simulink model "Copy_of_VTOLTiltrotor"  (R2024a)
settings: configuration reference "VTOLConfiguration" (kept outside this file)
undefined symbols (not defined in the file): airspeed, Battery, BCE12, BCE_Set_init, BMS_Controller_State, C, Cell10_P, Cell11_P, Cell12_P, Cell1_N, Cell1_P, Cell2_P, Cell3_P, Cell4_P, Cell5_P, Cell6_P, Cell7_P, Cell8_P, Cell9_P, Cell_Temperatures, Cell_Voltages, Charging_State, CityMission, control, controlParams, ControlSampleTime, CriticalTiltAngle, currentFactor, CV_Gain, ddx, ddy, ddz, Device_01, DiscIntNeverNeededParam, dx, dy, dz, Earth, env, F, F28379D_ADC_MaxCount, F28379D_ADC_Vmax, FixedWingMission, flightState, Foc_Ki_IxTcpu, Foc_Ki_S, Foc_Kp_I, Foc_Kp_S, fractalcoef, FSState, FWControlParams, HoverMission, I_cc, Ia_offset, Ib_offset, iniRoll, initPitch, iniYaw, IO334, IO334_DAC_Vmax ... (+55)
libraries: slrealtimeethercatlib x109, simulink x81, fl_lib x65, slpidlib x49, mcbcontrolslib x48, nesl_utility x43, speedgoatlib_hdlCoder_IO3xx x31, canmsglib x17, slrealtimeutilitieslib x13, mcbhdlplantlib x13, speedgoatlib_IO611 x12, dspstat3 x12
(part 5 of 20)

== system Copy_of_VTOLTiltrotor/Motor Control/Controller1/Controller_MIL ==
  Iab : Inport
  QAE_MIL_fbk : Inport  Port=2
  EnablePWM : Inport  Port=3
  Closed_Loop_FOC : Inport  Port=4
  Speed_CMD_RPM : Inport  Port=5
  Controller_Parameters : Inport  Port=6
  Bus Creator : BusCreator  Inputs=5
  Bus Selector : BusSelector  OutputSignals=Ia_offset,Ib_offset,Kp_S,Ki_S,Kp_I,Ki_IxTcpu
  Constant : Constant  Value=0  OutDataTypeStr=single  SampleTime=Ts_CPU
  Constant4 : Constant
  Data Type Conversion : DataTypeConversion  SaturateOnIntegerOverflow=off  RndMeth=Floor
  Data Type Conversion1 : DataTypeConversion  OutDataTypeStr=double  SaturateOnIntegerOverflow=off  RndMeth=Floor
  Data Type Conversion2 : DataTypeConversion  OutDataTypeStr=boolean  SaturateOnIntegerOverflow=off  RndMeth=Floor
  Data Type Conversion4 : DataTypeConversion  OutDataTypeStr=boolean  SaturateOnIntegerOverflow=off  RndMeth=Floor
  Data Type Conversion6 : DataTypeConversion  OutDataTypeStr=uint16  RndMeth=Simplest  SaturateOnIntegerOverflow=off
  F28379D ADC : Subsystem
  F28379D Firmware : Subsystem
  IO334 DAC : Subsystem
  Mux : Mux  Inputs=3
  PWM Generation : pwm_cpulib/PWM Generation  f_FPGA=f_FPGA  n_channels=3  sel_scaling=CPU  protection_param=A/B are forced off when A/B are on.  deadband_sec=0  natural_update=At period starts  delay=0  trigger_duration_sec=[1e-6]  trigger_period_start=off  trigger_half_of_the_period=off  trigger_a_on=off  trigger_a_off=off  trigger_b_on=off  trigger_b_off=off  bit_width_pwm_gen=24  invert_a=off  invert_b=off  invert_c=off
      settings: SourceProductName=PWM CPU Library
  PWM Periods : Constant  Value=[1/PWM_frequency 1/PWM_frequency 1/PWM_frequency]  OutDataTypeStr=double  SampleTime=-1
  Rate Transition1 : RateTransition  OutPortSampleTime=Ts_speed
  Rate Transition12 : RateTransition  OutPortSampleTime=Ts_UI
  Rate Transition{2,4..9} (7 alike) : RateTransition  OutPortSampleTime=Ts_CPU
  Rate Transition3 : RateTransition  OutPortSampleTime=Ts_speed
  bias1 : Constant  OutDataTypeStr=boolean  SampleTime=Ts_CPU
  bias3 : Constant  Value=0  OutDataTypeStr=boolean  SampleTime=Ts_CPU
  Simu_config : Outport
  Controller_fbk : Outport  Port=2
  wires:
  bias1/1 -> Bus Creator/1  "PCIe_RC_or_TTL"
  Bus Creator/1 -> Simu_config/1
  Constant4/1 -> Data Type Conversion6/1
  Data Type Conversion/1 -> Bus Creator/4  "PCIe_PWM_Enable"
  Iab/1 -> IO334 DAC/1(Iab)
  IO334 DAC/1(Iab_IO334DAC) -> F28379D ADC/1(Iab_IO334V)  "IabV"
  F28379D ADC/1(Ia_ADC) -> F28379D Firmware/1(Ia_ADC)
  F28379D ADC/2(Ib_ADC) -> F28379D Firmware/2(Ib_ADC)
  QAE_MIL_fbk/1 -> F28379D Firmware/5(QEP_Position_Count)
  Data Type Conversion6/1 -> F28379D Firmware/6(QEP_Index_Latch)
  Bus Selector/3 -> Rate Transition3/1  "<Kp_S>"
  F28379D Firmware/2(PWM_Enable) -> Data Type Conversion/1
  Data Type Conversion2/1 -> F28379D Firmware/11(EnablePWM)
  Data Type Conversion4/1 -> F28379D Firmware/10(EnClosedLoop)
  Bus Selector/4 -> Rate Transition1/1  "<Ki_S>"
  Closed_Loop_FOC/1 -> Rate Transition4/1
  Controller_Parameters/1 -> Bus Selector/1
  Bus Selector/1 -> Rate Transition5/1  "<Ia_offset>"
  Bus Selector/2 -> Rate Transition6/1  "<Ib_offset>"
  Bus Selector/5 -> Rate Transition8/1  "<Kp_I>"
  Bus Selector/6 -> Rate Transition9/1  "<Ki_IxTcpu>"
  EnablePWM/1 -> Rate Transition7/1
  Mux/1 -> Rate Transition12/1
  F28379D Firmware/3(Fbk_CAN) -> Mux/1
  Speed_CMD_RPM/1 -> Rate Transition2/1
  Rate Transition3/1 -> F28379D Firmware/8(Kp_S)
  Rate Transition1/1 -> F28379D Firmware/9(Ki_S)
  Rate Transition5/1 -> F28379D Firmware/3(IaOffset)
  Rate Transition6/1 -> F28379D Firmware/4(IbOffset)
  Rate Transition4/1 -> Data Type Conversion4/1
  Rate Transition7/1 -> Data Type Conversion2/1
  Rate Transition8/1 -> F28379D Firmware/12(Kp_i)
  Rate Transition9/1 -> F28379D Firmware/13(Ki_ixTcpu)
  Rate Transition12/1 -> Controller_fbk/1
  Constant/1 -> Mux/3
  Rate Transition2/1 -> F28379D Firmware/7(SpdCmdRPM), Mux/2
  bias3/1 -> Bus Creator/5  "PCIe_Protocol"
  PWM Periods/1 -> PWM Generation/1
  PWM Generation/1 -> Bus Creator/2  "PCIe_PWM_Config"
  PWM Generation/2 -> Bus Creator/3  "PCIe_PWM_Runtime"
  Data Type Conversion1/1 -> PWM Generation/2
  F28379D Firmware/1(ModWave) -> Data Type Conversion1/1

== system Copy_of_VTOLTiltrotor/Motor Control/Controller2/Controller_MIL ==
  Iab : Inport
  QAE_MIL_fbk : Inport  Port=2
  EnablePWM : Inport  Port=3
  Closed_Loop_FOC : Inport  Port=4
  Speed_CMD_RPM : Inport  Port=5
  Controller_Parameters : Inport  Port=6
  Bus Creator : BusCreator  Inputs=5
  Bus Selector : BusSelector  OutputSignals=Ia_offset,Ib_offset,Kp_S,Ki_S,Kp_I,Ki_IxTcpu
  Constant : Constant  Value=0  OutDataTypeStr=single  SampleTime=Ts_CPU
  Constant4 : Constant
  Data Type Conversion : DataTypeConversion  SaturateOnIntegerOverflow=off  RndMeth=Floor
  Data Type Conversion1 : DataTypeConversion  OutDataTypeStr=double  SaturateOnIntegerOverflow=off  RndMeth=Floor
  Data Type Conversion2 : DataTypeConversion  OutDataTypeStr=boolean  SaturateOnIntegerOverflow=off  RndMeth=Floor
  Data Type Conversion4 : DataTypeConversion  OutDataTypeStr=boolean  SaturateOnIntegerOverflow=off  RndMeth=Floor
  Data Type Conversion6 : DataTypeConversion  OutDataTypeStr=uint16  RndMeth=Simplest  SaturateOnIntegerOverflow=off
  F28379D ADC : Subsystem
  F28379D Firmware : Subsystem
  IO334 DAC : Subsystem
  Mux : Mux  Inputs=3
  PWM Generation : pwm_cpulib/PWM Generation  f_FPGA=f_FPGA  n_channels=3  sel_scaling=CPU  protection_param=A/B are forced off when A/B are on.  deadband_sec=0  natural_update=At period starts  delay=0  trigger_duration_sec=[1e-6]  trigger_period_start=off  trigger_half_of_the_period=off  trigger_a_on=off  trigger_a_off=off  trigger_b_on=off  trigger_b_off=off  bit_width_pwm_gen=24  invert_a=off  invert_b=off  invert_c=off
      settings: SourceProductName=PWM CPU Library
  PWM Periods : Constant  Value=[1/PWM_frequency 1/PWM_frequency 1/PWM_frequency]  OutDataTypeStr=double  SampleTime=-1
  Rate Transition1 : RateTransition  OutPortSampleTime=Ts_speed
  Rate Transition12 : RateTransition  OutPortSampleTime=Ts_UI
  Rate Transition{2,4..9} (7 alike) : RateTransition  OutPortSampleTime=Ts_CPU
  Rate Transition3 : RateTransition  OutPortSampleTime=Ts_speed
  bias1 : Constant  OutDataTypeStr=boolean  SampleTime=Ts_CPU
  bias3 : Constant  Value=0  OutDataTypeStr=boolean  SampleTime=Ts_CPU
  Simu_config : Outport
  Controller_fbk : Outport  Port=2
  wires:
  bias1/1 -> Bus Creator/1  "PCIe_RC_or_TTL"
  Bus Creator/1 -> Simu_config/1
  Constant4/1 -> Data Type Conversion6/1
  Data Type Conversion/1 -> Bus Creator/4  "PCIe_PWM_Enable"
  Iab/1 -> IO334 DAC/1(Iab)
  IO334 DAC/1(Iab_IO334DAC) -> F28379D ADC/1(Iab_IO334V)  "IabV"
  F28379D ADC/1(Ia_ADC) -> F28379D Firmware/1(Ia_ADC)
  F28379D ADC/2(Ib_ADC) -> F28379D Firmware/2(Ib_ADC)
  QAE_MIL_fbk/1 -> F28379D Firmware/5(QEP_Position_Count)
  Data Type Conversion6/1 -> F28379D Firmware/6(QEP_Index_Latch)
  Bus Selector/3 -> Rate Transition3/1  "<Kp_S>"
  F28379D Firmware/2(PWM_Enable) -> Data Type Conversion/1
  Data Type Conversion2/1 -> F28379D Firmware/11(EnablePWM)
  Data Type Conversion4/1 -> F28379D Firmware/10(EnClosedLoop)
  Bus Selector/4 -> Rate Transition1/1  "<Ki_S>"
  Closed_Loop_FOC/1 -> Rate Transition4/1
  Controller_Parameters/1 -> Bus Selector/1
  Bus Selector/1 -> Rate Transition5/1  "<Ia_offset>"
  Bus Selector/2 -> Rate Transition6/1  "<Ib_offset>"
  Bus Selector/5 -> Rate Transition8/1  "<Kp_I>"
  Bus Selector/6 -> Rate Transition9/1  "<Ki_IxTcpu>"
  EnablePWM/1 -> Rate Transition7/1
  Mux/1 -> Rate Transition12/1
  F28379D Firmware/3(Fbk_CAN) -> Mux/1
  Speed_CMD_RPM/1 -> Rate Transition2/1
  Rate Transition3/1 -> F28379D Firmware/8(Kp_S)
  Rate Transition1/1 -> F28379D Firmware/9(Ki_S)
  Rate Transition5/1 -> F28379D Firmware/3(IaOffset)
  Rate Transition6/1 -> F28379D Firmware/4(IbOffset)
  Rate Transition4/1 -> Data Type Conversion4/1
  Rate Transition7/1 -> Data Type Conversion2/1
  Rate Transition8/1 -> F28379D Firmware/12(Kp_i)
  Rate Transition9/1 -> F28379D Firmware/13(Ki_ixTcpu)
  Rate Transition12/1 -> Controller_fbk/1
  Constant/1 -> Mux/3
  Rate Transition2/1 -> F28379D Firmware/7(SpdCmdRPM), Mux/2
  bias3/1 -> Bus Creator/5  "PCIe_Protocol"
  PWM Periods/1 -> PWM Generation/1
  PWM Generation/1 -> Bus Creator/2  "PCIe_PWM_Config"
  PWM Generation/2 -> Bus Creator/3  "PCIe_PWM_Runtime"
  Data Type Conversion1/1 -> PWM Generation/2
  F28379D Firmware/1(ModWave) -> Data Type Conversion1/1

== system Copy_of_VTOLTiltrotor/Motor Control/Controller3/Controller_MIL ==
  Iab : Inport
  QAE_MIL_fbk : Inport  Port=2
  EnablePWM : Inport  Port=3
  Closed_Loop_FOC : Inport  Port=4
  Speed_CMD_RPM : Inport  Port=5
  Controller_Parameters : Inport  Port=6
  Bus Creator : BusCreator  Inputs=5
  Bus Selector : BusSelector  OutputSignals=Ia_offset,Ib_offset,Kp_S,Ki_S,Kp_I,Ki_IxTcpu
  Constant : Constant  Value=0  OutDataTypeStr=single  SampleTime=Ts_CPU
  Constant4 : Constant
  Data Type Conversion : DataTypeConversion  SaturateOnIntegerOverflow=off  RndMeth=Floor
  Data Type Conversion1 : DataTypeConversion  OutDataTypeStr=double  SaturateOnIntegerOverflow=off  RndMeth=Floor
  Data Type Conversion2 : DataTypeConversion  OutDataTypeStr=boolean  SaturateOnIntegerOverflow=off  RndMeth=Floor
  Data Type Conversion4 : DataTypeConversion  OutDataTypeStr=boolean  SaturateOnIntegerOverflow=off  RndMeth=Floor
  Data Type Conversion6 : DataTypeConversion  OutDataTypeStr=uint16  RndMeth=Simplest  SaturateOnIntegerOverflow=off
  F28379D ADC : Subsystem
  F28379D Firmware : Subsystem
  IO334 DAC : Subsystem
  Mux : Mux  Inputs=3
  PWM Generation : pwm_cpulib/PWM Generation  f_FPGA=f_FPGA  n_channels=3  sel_scaling=CPU  protection_param=A/B are forced off when A/B are on.  deadband_sec=0  natural_update=At period starts  delay=0  trigger_duration_sec=[1e-6]  trigger_period_start=off  trigger_half_of_the_period=off  trigger_a_on=off  trigger_a_off=off  trigger_b_on=off  trigger_b_off=off  bit_width_pwm_gen=24  invert_a=off  invert_b=off  invert_c=off
      settings: SourceProductName=PWM CPU Library
  PWM Periods : Constant  Value=[1/PWM_frequency 1/PWM_frequency 1/PWM_frequency]  OutDataTypeStr=double  SampleTime=-1
  Rate Transition1 : RateTransition  OutPortSampleTime=Ts_speed
  Rate Transition12 : RateTransition  OutPortSampleTime=Ts_UI
  Rate Transition{2,4..9} (7 alike) : RateTransition  OutPortSampleTime=Ts_CPU
  Rate Transition3 : RateTransition  OutPortSampleTime=Ts_speed
  bias1 : Constant  OutDataTypeStr=boolean  SampleTime=Ts_CPU
  bias3 : Constant  Value=0  OutDataTypeStr=boolean  SampleTime=Ts_CPU
  Simu_config : Outport
  Controller_fbk : Outport  Port=2
  wires:
  bias1/1 -> Bus Creator/1  "PCIe_RC_or_TTL"
  Bus Creator/1 -> Simu_config/1
  Constant4/1 -> Data Type Conversion6/1
  Data Type Conversion/1 -> Bus Creator/4  "PCIe_PWM_Enable"
  Iab/1 -> IO334 DAC/1(Iab)
  IO334 DAC/1(Iab_IO334DAC) -> F28379D ADC/1(Iab_IO334V)  "IabV"
  F28379D ADC/1(Ia_ADC) -> F28379D Firmware/1(Ia_ADC)
  F28379D ADC/2(Ib_ADC) -> F28379D Firmware/2(Ib_ADC)
  QAE_MIL_fbk/1 -> F28379D Firmware/5(QEP_Position_Count)
  Data Type Conversion6/1 -> F28379D Firmware/6(QEP_Index_Latch)
  Bus Selector/3 -> Rate Transition3/1  "<Kp_S>"
  F28379D Firmware/2(PWM_Enable) -> Data Type Conversion/1
  Data Type Conversion2/1 -> F28379D Firmware/11(EnablePWM)
  Data Type Conversion4/1 -> F28379D Firmware/10(EnClosedLoop)
  Bus Selector/4 -> Rate Transition1/1  "<Ki_S>"
  Closed_Loop_FOC/1 -> Rate Transition4/1
  Controller_Parameters/1 -> Bus Selector/1
  Bus Selector/1 -> Rate Transition5/1  "<Ia_offset>"
  Bus Selector/2 -> Rate Transition6/1  "<Ib_offset>"
  Bus Selector/5 -> Rate Transition8/1  "<Kp_I>"
  Bus Selector/6 -> Rate Transition9/1  "<Ki_IxTcpu>"
  EnablePWM/1 -> Rate Transition7/1
  Mux/1 -> Rate Transition12/1
  F28379D Firmware/3(Fbk_CAN) -> Mux/1
  Speed_CMD_RPM/1 -> Rate Transition2/1
  Rate Transition3/1 -> F28379D Firmware/8(Kp_S)
  Rate Transition1/1 -> F28379D Firmware/9(Ki_S)
  Rate Transition5/1 -> F28379D Firmware/3(IaOffset)
  Rate Transition6/1 -> F28379D Firmware/4(IbOffset)
  Rate Transition4/1 -> Data Type Conversion4/1
  Rate Transition7/1 -> Data Type Conversion2/1
  Rate Transition8/1 -> F28379D Firmware/12(Kp_i)
  Rate Transition9/1 -> F28379D Firmware/13(Ki_ixTcpu)
  Rate Transition12/1 -> Controller_fbk/1
  Constant/1 -> Mux/3
  Rate Transition2/1 -> F28379D Firmware/7(SpdCmdRPM), Mux/2
  bias3/1 -> Bus Creator/5  "PCIe_Protocol"
  PWM Periods/1 -> PWM Generation/1
  PWM Generation/1 -> Bus Creator/2  "PCIe_PWM_Config"
  PWM Generation/2 -> Bus Creator/3  "PCIe_PWM_Runtime"
  Data Type Conversion1/1 -> PWM Generation/2
  F28379D Firmware/1(ModWave) -> Data Type Conversion1/1

== system Copy_of_VTOLTiltrotor/Motor Control/Three-Phase PMSM Drive/PMSM and average inverter ==
  Simu_config : Inport
  V_dc : Inport  Port=2
  Fault : Inport  Port=3
  LdTrq/Spd : Inport  Port=4
  Add : Sum
  Bus Selector : BusSelector  OutputSignals=PCIe_PWM_Runtime
  Clarke Transform : mcbhdlplantlib/PMSM HDL/PMSM Electromagnetic/Clarke Transform  SystemSampleTime=-1  VariantActivationTime=update diagram  AllowFlexibleInterface=on  Latency=0  AutoFrameSizeCalculation=off
  Demux : Demux  Outputs=3
  Demux1 : Demux  Outputs=2
  Demux2 : Demux  Outputs=2
  Divide : Product  Inputs=*/
  Encoder Simulation : Subsystem
  Gain : Gain  Gain=-1
  Ideal Inverter : Subsystem
  Memory : Memory  InheritSampleTime=on
  Memory1 : Memory  InheritSampleTime=on
  Memory2 : Memory  InitialCondition=48  InheritSampleTime=on
  PMSM : Subsystem
  PMSM HDL Configuration : mcbhdlplantlib/PMSM Configuration  portConfig=Torque  Trq_N_mode=0  Ts=Ts_CPU  Pp=Maxon_645604_Np  Rs=Maxon_645604_Rs  Ld=Maxon_645604_Ld  Lq=Maxon_645604_Lq  lambda_pm=Maxon_645604_lambda_pm  J=Maxon_645604_J  B=Maxon_645604_ViscousF*100  f=Maxon_645604_StaticF
  Park Transform : mcbcontrolslib/Park Transform  PhaseInput=Two inputs  AxisAlignment=D-axis  ThetaInput=Sine and Cosine electrical position  AngleInput=Radians  N_points=1024
  Product : Product
  Product1 : Product
  Runtime to DC : Subsystem
  Selec Angle1 : Selector  InputPortWidth=14  IndexOptions=Index vector (dialog)  Indices=[10]  OutputSizes=1
  Selec Angle2 : Selector  InputPortWidth=14  IndexOptions=Index vector (dialog)  Indices=[13 14]  OutputSizes=1
  Selec Angle3 : Selector  InputPortWidth=14  IndexOptions=Index vector (dialog)  Indices=[4 5]  OutputSizes=1
  Terminator : Terminator
  Terminator1 : Terminator
  Terminator2 : Terminator
  Ia : Outport
  Ib : Outport  Port=2
  Ic : Outport  Port=3
  Motor_Spd : Outport  Port=4
  Motor_Angle : Outport  Port=5
  QAE_Pos_C : Outport  Port=6
  tag scope: Idc1=global
  wires:
  PMSM/4(RotorMechSpd) -> Motor_Spd/1
  Demux/2 -> Ib/1
  Selec Angle1/1 -> Motor_Angle/1, Encoder Simulation/1(Theta_m)
  Demux/3 -> Ic/1
  LdTrq/Spd/1 -> PMSM/3(LdTrq / Spd)
  PMSM HDL Configuration/1 -> PMSM/1(Config)
  PMSM/2(PhaseCurr) -> Demux/1
  Demux/1 -> Ia/1
  Ideal Inverter/1(Vabc) -> Clarke Transform/1, PMSM/2(PhaseVolt abc)
  V_dc/1 -> Ideal Inverter/1(V_DC)
  Simu_config/1 -> Bus Selector/1
  Fault/1 -> Terminator/1
  Encoder Simulation/1(QEP_Position_Count) -> QAE_Pos_C/1
  PMSM/3(Torque) -> Terminator1/1
  PMSM/5(RotorElecAngle) -> Terminator2/1
  PMSM/1(Info) -> Selec Angle3/1, Selec Angle2/1, Selec Angle1/1
  Bus Selector/1 -> Runtime to DC/1(PWM_Runtime)  "<PCIe_PWM_Runtime>"
  Runtime to DC/1(Duty Cycle abc) -> Ideal Inverter/2(Duty Cycle abc)
  Clarke Transform/1 -> Park Transform/1
  Clarke Transform/2 -> Park Transform/2
  Demux1/1 -> Park Transform/3
  Demux1/2 -> Park Transform/4
  Selec Angle2/1 -> Memory1/1
  Park Transform/1 -> Product/1
  Park Transform/2 -> Product1/1
  Selec Angle3/1 -> Memory/1
  Demux2/1 -> Product/2
  Demux2/2 -> Product1/2
  Product/1 -> Add/1
  Product1/1 -> Add/2
  Add/1 -> Divide/1
  [Voltage] -> Memory2/1
  Divide/1 -> Gain/1
  Memory/1 -> Demux2/1
  Memory1/1 -> Demux1/1
  Memory2/1 -> Divide/2
  Gain/1 -> [Idc1]

== system Copy_of_VTOLTiltrotor/Motor Control/Three-Phase PMSM Drive/PMSM and inverter with switching dynamics ==
  Simu_config : Inport
  V_dc : Inport  Port=2
  Fault : Inport  Port=3
  LdTrq/Spd : Inport  Port=4
  Bus Selector : BusSelector  OutputSignals=PCIe_RC_or_TTL,PCIe_PWM_Config,PCIe_PWM_Runtime,PCIe_PWM_Enable,PCIe_Protocol
  DAC Config : Subsystem
  Encoder Simulation : Subsystem
  Motor Connection : Constant  OutDataTypeStr=boolean
  PMSM HDL Configuration : mcbhdlplantlib/PMSM Configuration  portConfig=Torque  Trq_N_mode=0  Ts=Ts_UI  Pp=Maxon_645604_Np  Rs=Maxon_645604_Rs  Ld=Maxon_645604_Ld  Lq=Maxon_645604_Lq  lambda_pm=Maxon_645604_lambda_pm  J=Maxon_645604_J  B=Maxon_645604_ViscousF*100  f=Maxon_645604_StaticF
  PMSM_3P2L_Inverter_Plant_TBR : Subsystem
      mask Display: disp('Plant Bitstream Block')
  Quadrature Encoder : quadrature_cpulib/Quadrature Encoder  FPGA_freq=f_FPGA  n_channels=[1]  sel_scaling=FPGA  useSpeed=off  usePosition=on  numOfSlots=Maxon_Mile_Nslits  sigAswitchOn=[180]  sigBswitchOff=[90]  sigBswitchOn=[270]  sigAdismissEn=off  sigAdismissSingle=on  sigAdismissHigh=on  sigBdismissEn=off  sigBdismissSingle=on  sigBdismissHigh=on
      settings: SourceProductName=Quadrature CPU Library
  Resolver Encoder : resolver_cpulib/Resolver Encoder  Ts=Ts_UI  ts_resolver=ts_FPGA_mdl  sel_scaling=FPGA  useSpeed=on  usePosition=off  pole_pairs=1  gain_dynamic=off  gainVector=[1, 1, 1, 1]  offset_dynamic=off  offsetVector=[0, 0, 0, 0]  exct_freq=2  angle_offset=0  exct_amplitude=10  position_init_enb=off  rotor_position=90  int_exct_enb=on  exct_out_enb=on  phase_delay=0  time_step_delay=0  adcRange=2.5  dacRange=2.5
      settings: SourceProductName=Resolver CPU Library
  Terminator{21,32..34,40..41,45..46} (8 alike) : Terminator
  Ia : Outport
  Ib : Outport  Port=2
  Ic : Outport  Port=3
  Motor_Spd : Outport  Port=4
  Motor_Angle : Outport  Port=5
  QAE_Pos_C : Outport  Port=6
  wires:
  PMSM_3P2L_Inverter_Plant_TBR/10(PCIe_Rsvl_excitation_neg) -> Terminator33/1
  DAC Config/1(I_DAC_gain) -> PMSM_3P2L_Inverter_Plant_TBR/13(PCIe_Iabc_DAC_gain)
  DAC Config/3(DAC_reset) -> PMSM_3P2L_Inverter_Plant_TBR/15(PCIe_DAC_reset)
  PMSM_3P2L_Inverter_Plant_TBR/7(PCIe_Motor_ElecAngle) -> Terminator21/1
  PMSM_3P2L_Inverter_Plant_TBR/12(PCIe_Rsvl_cos_neg) -> Terminator41/1
  PMSM_3P2L_Inverter_Plant_TBR/13(PCIe_Resolver_Out) -> Terminator40/1
  V_dc/1 -> PMSM_3P2L_Inverter_Plant_TBR/6(PCIe_V_dc)
  PMSM_3P2L_Inverter_Plant_TBR/8(PCIe_Motor_Trq) -> Terminator46/1
  Resolver Encoder/1 -> PMSM_3P2L_Inverter_Plant_TBR/12(PCIe_Resolver_Config)
  PMSM_3P2L_Inverter_Plant_TBR/4(PCIe_Idc) -> Terminator45/1
  Quadrature Encoder/1 -> PMSM_3P2L_Inverter_Plant_TBR/11(PCIe_QAE_Config)
  Motor Connection/1 -> PMSM_3P2L_Inverter_Plant_TBR/10(PCIe_Motor_Connection)
  PMSM_3P2L_Inverter_Plant_TBR/9(PCIe_Rsvl_excitation_pos) -> Terminator32/1
  Fault/1 -> PMSM_3P2L_Inverter_Plant_TBR/7(PCIe_Fault)
  PMSM_3P2L_Inverter_Plant_TBR/11(PCIe_Rsvl_sin_neg) -> Terminator34/1
  DAC Config/2(I_DAC_Current) -> PMSM_3P2L_Inverter_Plant_TBR/14(PCIe_Iabc_DAC_bias)
  PMSM HDL Configuration/1 -> PMSM_3P2L_Inverter_Plant_TBR/9(PCIe_Motor_Config)
  Simu_config/1 -> Bus Selector/1
  Bus Selector/4 -> PMSM_3P2L_Inverter_Plant_TBR/4(PCIe_PWM_Enable)  "<PCIe_PWM_Enable>"
  Bus Selector/5 -> PMSM_3P2L_Inverter_Plant_TBR/5(PCIe_Protocol)  "<PCIe_Protocol>"
  Bus Selector/1 -> PMSM_3P2L_Inverter_Plant_TBR/1(PCIe_RC_or_TTL)  "<PCIe_RC_or_TTL>"
  LdTrq/Spd/1 -> PMSM_3P2L_Inverter_Plant_TBR/8(PCIe_LdTrq/Spd)
  PMSM_3P2L_Inverter_Plant_TBR/3(PCIe_Ic) -> Ic/1
  PMSM_3P2L_Inverter_Plant_TBR/6(PCIe_Motor_Angle) -> Motor_Angle/1, Encoder Simulation/1(Theta_m)
  PMSM_3P2L_Inverter_Plant_TBR/5(PCIe_Motor_Spd) -> Motor_Spd/1
  PMSM_3P2L_Inverter_Plant_TBR/2(PCIe_Ib) -> Ib/1
  Encoder Simulation/1(QEP_Position_Count) -> QAE_Pos_C/1
  PMSM_3P2L_Inverter_Plant_TBR/1(PCIe_Ia) -> Ia/1
  Bus Selector/3 -> PMSM_3P2L_Inverter_Plant_TBR/3(PCIe_PWM_Runtime)  "<PCIe_PWM_Runtime>"
  Bus Selector/2 -> PMSM_3P2L_Inverter_Plant_TBR/2(PCIe_PWM_Config)  "<PCIe_PWM_Config>"

== system Copy_of_VTOLTiltrotor/Motor Control/Three-Phase PMSM Drive1/PMSM and average inverter ==
  Simu_config : Inport
  V_dc : Inport  Port=2
  Fault : Inport  Port=3
  LdTrq/Spd : Inport  Port=4
  Add : Sum
  Bus Selector : BusSelector  OutputSignals=PCIe_PWM_Runtime
  Clarke Transform : mcbhdlplantlib/PMSM HDL/PMSM Electromagnetic/Clarke Transform  SystemSampleTime=-1  VariantActivationTime=update diagram  AllowFlexibleInterface=on  Latency=0  AutoFrameSizeCalculation=off
  Demux : Demux  Outputs=3
  Demux1 : Demux  Outputs=2
  Demux2 : Demux  Outputs=2
  Divide : Product  Inputs=*/
  Encoder Simulation : Subsystem
  Gain : Gain  Gain=-1
  Ideal Inverter : Subsystem
  Memory : Memory  InheritSampleTime=on
  Memory1 : Memory  InheritSampleTime=on
  Memory2 : Memory  InitialCondition=48  InheritSampleTime=on
  PMSM : Subsystem
  PMSM HDL Configuration : mcbhdlplantlib/PMSM Configuration  portConfig=Torque  Trq_N_mode=0  Ts=Ts_CPU  Pp=Maxon_645604_Np  Rs=Maxon_645604_Rs  Ld=Maxon_645604_Ld  Lq=Maxon_645604_Lq  lambda_pm=Maxon_645604_lambda_pm  J=Maxon_645604_J  B=Maxon_645604_ViscousF*100  f=Maxon_645604_StaticF
  Park Transform : mcbcontrolslib/Park Transform  PhaseInput=Two inputs  AxisAlignment=D-axis  ThetaInput=Sine and Cosine electrical position  AngleInput=Radians  N_points=1024
  Product : Product
  Product1 : Product
  Runtime to DC : Subsystem
  Selec Angle1 : Selector  InputPortWidth=14  IndexOptions=Index vector (dialog)  Indices=[10]  OutputSizes=1
  Selec Angle2 : Selector  InputPortWidth=14  IndexOptions=Index vector (dialog)  Indices=[13 14]  OutputSizes=1
  Selec Angle3 : Selector  InputPortWidth=14  IndexOptions=Index vector (dialog)  Indices=[4 5]  OutputSizes=1
  Terminator : Terminator
  Terminator1 : Terminator
  Terminator2 : Terminator
  Ia : Outport
  Ib : Outport  Port=2
  Ic : Outport  Port=3
  Motor_Spd : Outport  Port=4
  Motor_Angle : Outport  Port=5
  QAE_Pos_C : Outport  Port=6
  tag scope: Idc2=global
  wires:
  PMSM/4(RotorMechSpd) -> Motor_Spd/1
  Demux/2 -> Ib/1
  Selec Angle1/1 -> Motor_Angle/1, Encoder Simulation/1(Theta_m)
  Demux/3 -> Ic/1
  LdTrq/Spd/1 -> PMSM/3(LdTrq / Spd)
  PMSM HDL Configuration/1 -> PMSM/1(Config)
  PMSM/2(PhaseCurr) -> Demux/1
  Demux/1 -> Ia/1
  Ideal Inverter/1(Vabc) -> Clarke Transform/1, PMSM/2(PhaseVolt abc)
  V_dc/1 -> Ideal Inverter/1(V_DC)
  Simu_config/1 -> Bus Selector/1
  Fault/1 -> Terminator/1
  Encoder Simulation/1(QEP_Position_Count) -> QAE_Pos_C/1
  PMSM/3(Torque) -> Terminator1/1
  PMSM/5(RotorElecAngle) -> Terminator2/1
  PMSM/1(Info) -> Selec Angle3/1, Selec Angle2/1, Selec Angle1/1
  Bus Selector/1 -> Runtime to DC/1(PWM_Runtime)  "<PCIe_PWM_Runtime>"
  Runtime to DC/1(Duty Cycle abc) -> Ideal Inverter/2(Duty Cycle abc)
  Clarke Transform/1 -> Park Transform/1
  Clarke Transform/2 -> Park Transform/2
  Demux1/1 -> Park Transform/3
  Demux1/2 -> Park Transform/4
  Selec Angle2/1 -> Memory1/1
  Park Transform/1 -> Product/1
  Park Transform/2 -> Product1/1
  Selec Angle3/1 -> Memory/1
  Demux2/1 -> Product/2
  Demux2/2 -> Product1/2
  Product/1 -> Add/1
  Product1/1 -> Add/2
  Add/1 -> Divide/1
  [Voltage] -> Memory2/1
  Divide/1 -> Gain/1
  Memory/1 -> Demux2/1
  Memory1/1 -> Demux1/1
  Memory2/1 -> Divide/2
  Gain/1 -> [Idc2]

== system Copy_of_VTOLTiltrotor/Motor Control/Three-Phase PMSM Drive2/PMSM and average inverter ==
  Simu_config : Inport
  V_dc : Inport  Port=2
  Fault : Inport  Port=3
  LdTrq/Spd : Inport  Port=4
  Add : Sum
  Bus Selector : BusSelector  OutputSignals=PCIe_PWM_Runtime
  Clarke Transform : mcbhdlplantlib/PMSM HDL/PMSM Electromagnetic/Clarke Transform  SystemSampleTime=-1  VariantActivationTime=update diagram  AllowFlexibleInterface=on  Latency=0  AutoFrameSizeCalculation=off
  Demux : Demux  Outputs=3
  Demux1 : Demux  Outputs=2
  Demux2 : Demux  Outputs=2
  Divide : Product  Inputs=*/
  Encoder Simulation : Subsystem
  Gain : Gain  Gain=-1
  Ideal Inverter : Subsystem
  Memory : Memory  InheritSampleTime=on
  Memory1 : Memory  InheritSampleTime=on
  Memory2 : Memory  InitialCondition=48  InheritSampleTime=on
  PMSM : Subsystem
  PMSM HDL Configuration : mcbhdlplantlib/PMSM Configuration  portConfig=Torque  Trq_N_mode=0  Ts=Ts_CPU  Pp=Maxon_645604_Np  Rs=Maxon_645604_Rs  Ld=Maxon_645604_Ld  Lq=Maxon_645604_Lq  lambda_pm=Maxon_645604_lambda_pm  J=Maxon_645604_J  B=Maxon_645604_ViscousF*100  f=Maxon_645604_StaticF
  Park Transform : mcbcontrolslib/Park Transform  PhaseInput=Two inputs  AxisAlignment=D-axis  ThetaInput=Sine and Cosine electrical position  AngleInput=Radians  N_points=1024
  Product : Product
  Product1 : Product
  Runtime to DC : Subsystem
  Selec Angle1 : Selector  InputPortWidth=14  IndexOptions=Index vector (dialog)  Indices=[10]  OutputSizes=1
  Selec Angle2 : Selector  InputPortWidth=14  IndexOptions=Index vector (dialog)  Indices=[13 14]  OutputSizes=1
  Selec Angle3 : Selector  InputPortWidth=14  IndexOptions=Index vector (dialog)  Indices=[4 5]  OutputSizes=1
  Terminator : Terminator
  Terminator1 : Terminator
  Terminator2 : Terminator
  Ia : Outport
  Ib : Outport  Port=2
  Ic : Outport  Port=3
  Motor_Spd : Outport  Port=4
  Motor_Angle : Outport  Port=5
  QAE_Pos_C : Outport  Port=6
  tag scope: Idc3=global
  wires:
  PMSM/4(RotorMechSpd) -> Motor_Spd/1
  Demux/2 -> Ib/1
  Selec Angle1/1 -> Motor_Angle/1, Encoder Simulation/1(Theta_m)
  Demux/3 -> Ic/1
  LdTrq/Spd/1 -> PMSM/3(LdTrq / Spd)
  PMSM HDL Configuration/1 -> PMSM/1(Config)
  PMSM/2(PhaseCurr) -> Demux/1
  Demux/1 -> Ia/1
  Ideal Inverter/1(Vabc) -> Clarke Transform/1, PMSM/2(PhaseVolt abc)
  V_dc/1 -> Ideal Inverter/1(V_DC)
  Simu_config/1 -> Bus Selector/1
  Fault/1 -> Terminator/1
  Encoder Simulation/1(QEP_Position_Count) -> QAE_Pos_C/1
  PMSM/3(Torque) -> Terminator1/1
  PMSM/5(RotorElecAngle) -> Terminator2/1
  PMSM/1(Info) -> Selec Angle3/1, Selec Angle2/1, Selec Angle1/1
  Bus Selector/1 -> Runtime to DC/1(PWM_Runtime)  "<PCIe_PWM_Runtime>"
  Runtime to DC/1(Duty Cycle abc) -> Ideal Inverter/2(Duty Cycle abc)
  Clarke Transform/1 -> Park Transform/1
  Clarke Transform/2 -> Park Transform/2
  Demux1/1 -> Park Transform/3
  Demux1/2 -> Park Transform/4
  Selec Angle2/1 -> Memory1/1
  Park Transform/1 -> Product/1
  Park Transform/2 -> Product1/1
  Selec Angle3/1 -> Memory/1
  Demux2/1 -> Product/2
  Demux2/2 -> Product1/2
  Product/1 -> Add/1
  Product1/1 -> Add/2
  Add/1 -> Divide/1
  [Voltage] -> Memory2/1
  Divide/1 -> Gain/1
  Memory/1 -> Demux2/1
  Memory1/1 -> Demux1/1
  Memory2/1 -> Divide/2
  Gain/1 -> [Idc3]

== system Copy_of_VTOLTiltrotor/Motor Control/Three-Phase PMSM Drive3/PMSM and average inverter ==
  Simu_config : Inport
  V_dc : Inport  Port=2
  Fault : Inport  Port=3
  LdTrq/Spd : Inport  Port=4
  Add : Sum
  Bus Selector : BusSelector  OutputSignals=PCIe_PWM_Runtime
  Clarke Transform : mcbhdlplantlib/PMSM HDL/PMSM Electromagnetic/Clarke Transform  SystemSampleTime=-1  VariantActivationTime=update diagram  AllowFlexibleInterface=on  Latency=0  AutoFrameSizeCalculation=off
  Demux : Demux  Outputs=3
  Demux1 : Demux  Outputs=2
  Demux2 : Demux  Outputs=2
  Divide : Product  Inputs=*/
  Encoder Simulation : Subsystem
  Gain : Gain  Gain=-1
  Ideal Inverter : Subsystem
  Memory : Memory  InheritSampleTime=on
  Memory1 : Memory  InheritSampleTime=on
  Memory2 : Memory  InitialCondition=48  InheritSampleTime=on
  PMSM : Subsystem
  PMSM HDL Configuration : mcbhdlplantlib/PMSM Configuration  portConfig=Torque  Trq_N_mode=0  Ts=Ts_CPU  Pp=Maxon_645604_Np  Rs=Maxon_645604_Rs  Ld=Maxon_645604_Ld  Lq=Maxon_645604_Lq  lambda_pm=Maxon_645604_lambda_pm  J=Maxon_645604_J  B=Maxon_645604_ViscousF*100  f=Maxon_645604_StaticF
  Park Transform : mcbcontrolslib/Park Transform  PhaseInput=Two inputs  AxisAlignment=D-axis  ThetaInput=Sine and Cosine electrical position  AngleInput=Radians  N_points=1024
  Product : Product
  Product1 : Product
  Runtime to DC : Subsystem
  Selec Angle1 : Selector  InputPortWidth=14  IndexOptions=Index vector (dialog)  Indices=[10]  OutputSizes=1
  Selec Angle2 : Selector  InputPortWidth=14  IndexOptions=Index vector (dialog)  Indices=[13 14]  OutputSizes=1
  Selec Angle3 : Selector  InputPortWidth=14  IndexOptions=Index vector (dialog)  Indices=[4 5]  OutputSizes=1
  Terminator : Terminator
  Terminator1 : Terminator
  Terminator2 : Terminator
  Ia : Outport
  Ib : Outport  Port=2
  Ic : Outport  Port=3
  Motor_Spd : Outport  Port=4
  Motor_Angle : Outport  Port=5
  QAE_Pos_C : Outport  Port=6
  tag scope: Idc4=global
  wires:
  PMSM/4(RotorMechSpd) -> Motor_Spd/1
  Demux/2 -> Ib/1
  Selec Angle1/1 -> Motor_Angle/1, Encoder Simulation/1(Theta_m)
  Demux/3 -> Ic/1
  LdTrq/Spd/1 -> PMSM/3(LdTrq / Spd)
  PMSM HDL Configuration/1 -> PMSM/1(Config)
  PMSM/2(PhaseCurr) -> Demux/1
  Demux/1 -> Ia/1
  Ideal Inverter/1(Vabc) -> Clarke Transform/1, PMSM/2(PhaseVolt abc)
  V_dc/1 -> Ideal Inverter/1(V_DC)
  Simu_config/1 -> Bus Selector/1
  Fault/1 -> Terminator/1
  Encoder Simulation/1(QEP_Position_Count) -> QAE_Pos_C/1
  PMSM/3(Torque) -> Terminator1/1
  PMSM/5(RotorElecAngle) -> Terminator2/1
  PMSM/1(Info) -> Selec Angle3/1, Selec Angle2/1, Selec Angle1/1
  Bus Selector/1 -> Runtime to DC/1(PWM_Runtime)  "<PCIe_PWM_Runtime>"
  Runtime to DC/1(Duty Cycle abc) -> Ideal Inverter/2(Duty Cycle abc)
  Clarke Transform/1 -> Park Transform/1
  Clarke Transform/2 -> Park Transform/2
  Demux1/1 -> Park Transform/3
  Demux1/2 -> Park Transform/4
  Selec Angle2/1 -> Memory1/1
  Park Transform/1 -> Product/1
  Park Transform/2 -> Product1/1
  Selec Angle3/1 -> Memory/1
  Demux2/1 -> Product/2
  Demux2/2 -> Product1/2
  Product/1 -> Add/1
  Product1/1 -> Add/2
  Add/1 -> Divide/1
  [Voltage] -> Memory2/1
  Divide/1 -> Gain/1
  Memory/1 -> Demux2/1
  Memory1/1 -> Demux1/1
  Memory2/1 -> Divide/2
  Gain/1 -> [Idc4]

== system Copy_of_VTOLTiltrotor/Visualization/Photorealistic/Prepare UAV Data ==
  UAVState : Inport
  Bus Selector1 : BusSelector  OutputSignals=x,y,z,yaw,pitch,roll
  Gain{,1..3} (4 alike) : Gain  Gain=-1
  Mux : Mux  Inputs=3
  Mux1 : Mux  Inputs=3
  Translation : Outport
  Rotation : Outport  Port=2
  wires:
  UAVState/1 -> Bus Selector1/1
  Mux/1 -> Translation/1
  Mux1/1 -> Rotation/1  "EulerZYX"
  Bus Selector1/4 -> Gain3/1  "<yaw>"
  Bus Selector1/5 -> Gain2/1  "<pitch>"
  Bus Selector1/6 -> Mux1/3  "<roll>"
  Bus Selector1/3 -> Gain/1  "<z>"
  Bus Selector1/2 -> Gain1/1  "<y>"
  Bus Selector1/1 -> Mux/1  "<x>"
  Gain/1 -> Mux/3
  Gain1/1 -> Mux/2
  Gain2/1 -> Mux1/2
  Gain3/1 -> Mux1/1

== system Copy_of_VTOLTiltrotor/Visualization/Visualization/Subsystem ==
  <Xe> : Inport
  <q> : Inport  Port=2
  RotorA : Inport  Port=3
  RotorB : Inport  Port=4
  Constant : Constant  Value=0
  Constant1 : Constant  Value=0
  Gain : Gain  Gain=0
  Gain1 : Gain  Gain=-1
  Gain2 : Gain  Gain=-1
  MATLAB System : MATLABSystem  System=exampleHelperTiltRotorAnimator  SampleTime=0.05
      mask Type: exampleHelperTiltRotorAnimator
      mask Display:
      | disp('exampleHelperTiltRotorAnimator');
      | port_label('input',1,'position');
      | port_label('input',2,'orientation');
      | port_label('input',3,'rotorAngles');
  Mux : Mux
  Reshape : Reshape  OutputDimensionality=Customize  OutputDimensions=[1,4]
  Reshape1 : Reshape  OutputDimensionality=Customize  OutputDimensions=[1,4]
  Reshape2 : Reshape  OutputDimensionality=Customize  OutputDimensions=[1,3]
  wires:
  Gain1/1 -> Mux/1
  Constant1/1 -> Mux/4
  Gain2/1 -> Mux/2
  Reshape1/1 -> MATLAB System/3
  Mux/1 -> Reshape1/1
  RotorA/1 -> Gain1/1
  <Xe>/1 -> Gain/1
  Constant/1 -> Mux/3
  RotorB/1 -> Gain2/1
  <q>/1 -> Reshape/1
  Reshape2/1 -> MATLAB System/1
  Reshape/1 -> MATLAB System/2
  Gain/1 -> Reshape2/1

== system Copy_of_VTOLTiltrotor/Battery Management System/BMS/HIL/Cell Monitoring Unit ==
  Bal_Cmd_Controller : Inport
  Sensor_Values : Inport  Port=2
  Bal_Cmd : Outport
  Sensor Values : Outport  Port=2
  wires:
  Sensor_Values/1 -> Sensor Values/1
  Bal_Cmd_Controller/1 -> Bal_Cmd/1  "Bal_Cmd"

== system Copy_of_VTOLTiltrotor/Battery Management System/BMS/HIL/Controller ==
  Sensor_Values : Inport  OutDataTypeStr=Bus: Sensor_Values  BusOutputAsStruct=on
  State_Request : Inport  Port=2  OutDataTypeStr=Enum: SRE  PortDimensions=1
  CAN & LIN Setup : speedgoatlib_IO611/Legacy/CAN & LIN Setup  id=1  drvLtr=C:  PCISlot=-1  port1=CAN (HS/LS)  port2=CAN (HS/LS)  port3=Disable  port4=Disable  opModeCAN1=Highspeed (HS)  bdrCAN1=1 MBaud  usrBdrCAN1=[5, 1, 13, 2]  bdrFD1=5 MBaud  usrBdrFD1=[2, 1, 5, 2, 75, 5000]  stdAccMaskCAN1=[0, 0]  extAccMaskCAN1=[0, 0]  opModeCAN2=Highspeed (HS)  bdrCAN2=1 MBaud  usrBdrCAN2=[5, 1, 13, 2]  bdrFD2=5 MBaud  usrBdrFD2=[2, 1, 5, 2, 75, 5000]  stdAccMaskCAN2=[0, 0]  extAccMaskCAN2=[0, 0]  initStruct=[]  termStruct=[]  opModeLIN3=Master  bdrLIN3=19200  opModeLIN4=Master  bdrLIN4=19200  protl=IO611  qtyMod=1  chNo=[1, 2, 3, 4]  ptTypes=[1, 1, 2, 2]  isProtlFD=[0, 0]  protlHelpIdx=[0, 1, 0, 1]  isFDMod=1
      settings: SourceProductName=IO611
  Constant10 : Constant  Value=uint8(SRE.Charging)
  Constant7 : Constant  Value=zeros(1,Ns_Module)
  Constant8 : Constant  Value=uint8(SRE.Standby)
  Constant9 : Constant  Value=uint8(SRE.Driving)
  Data Type Conversion : DataTypeConversion  OutDataTypeStr=boolean  SaturateOnIntegerOverflow=off  RndMeth=Floor
  Multiport Switch : MultiPortSwitch  DataPortOrder=Specify indices  DataPortIndices={SRE.Standby, SRE.Driving, SRE.Charging}  SaturateOnIntegerOverflow=off  InputSameDT=off
  PLANT-Rx : Subsystem  TreatAsAtomicUnit=on
  PLANT-Tx : Subsystem
  Rate Transition : RateTransition  InitialCondition=struct('OverCurrent',0,'HighTemp',0,'LowTemp',0,'OverVolt',0,'UnderVolt',0)  OutPortSampleTime=ts_controller
  Rate Transition1 : RateTransition  InitialCondition=Charging_State.Init  OutPortSampleTime=ts_controller
  Rate Transition2 : RateTransition  InitialCondition=BMS_Controller_State.BMS_Idle  OutPortSampleTime=ts_controller
  Rate Transition3 : RateTransition  InitialCondition=[0, 0, 0]  OutPortSampleTime=ts_controller
  Rate Transition4 : RateTransition  InitialCondition=-100  OutPortSampleTime=ts_controller
  Rate Transition5 : RateTransition  InitialCondition=40  OutPortSampleTime=ts_controller
  Rate Transition6 : RateTransition  OutPortSampleTime=ts_controller
  Rate Transition7 : RateTransition  OutPortSampleTime=ts_controller
  BMS_Faults : Outport
  Charging_State : Outport  Port=2
  BMS_State : Outport  Port=3
  SOC : Outport  Port=4
  Discharge_Current_Limit : Outport  Port=5
  Charge_Current_Limit : Outport  Port=6
  Charge_Current_Req : Outport  Port=7
  Bal_Cmd : Outport  Port=8
  wires:
  Constant7/1 -> Rate Transition7/1  "Bal_Cmd"
  Constant9/1 -> Multiport Switch/3
  Constant10/1 -> Multiport Switch/4
  Constant8/1 -> Multiport Switch/2
  State_Request/1 -> Multiport Switch/1
  PLANT-Rx/1(BMS_Faults) -> Rate Transition/1
  PLANT-Rx/7(Charge_Current_Req) -> Rate Transition6/1
  PLANT-Rx/6(Charge_Current_Limit) -> Rate Transition5/1
  PLANT-Rx/5(Discharge_Current_Limit) -> Rate Transition4/1
  PLANT-Rx/4(SOC) -> Rate Transition3/1
  PLANT-Rx/3(BMS_State) -> Rate Transition2/1
  PLANT-Rx/2(Charging_State) -> Rate Transition1/1
  Rate Transition/1 -> BMS_Faults/1  "Faults"
  Rate Transition1/1 -> Charging_State/1  "Charging_State"
  Rate Transition2/1 -> BMS_State/1  "BMS_State"
  Rate Transition3/1 -> SOC/1  "SOC"
  Rate Transition4/1 -> Discharge_Current_Limit/1  "Discharge_Current_Limit"
  Rate Transition5/1 -> Charge_Current_Limit/1  "Charge_Current_Limit"
  Rate Transition6/1 -> Charge_Current_Req/1  "Charge_Current_Req"
  Data Type Conversion/1 -> Bal_Cmd/1
  Rate Transition7/1 -> Data Type Conversion/1  "Charge_Current_Req"
  Sensor_Values/1 -> PLANT-Tx/1(to_Controller)
  Multiport Switch/1 -> PLANT-Tx/2(to_Controller_SRE)  "SRE"

== system Copy_of_VTOLTiltrotor/Battery Management System/BMS/MIL/Cell Monitoring Unit ==
  Bal_Cmd_Controller : Inport
  Sensor_Values : Inport  Port=2
  Balancing_Circuit : Subsystem
  Feedback Unit : UnitDelay  InitialCondition=struct('Cell_Voltages',3.6*ones(1, Ns_Module*NumModules),'Cell_Temperatures',293.15*ones(1,Ns_Module*NumModules),'Pack_Current',0,'Pack_Voltage',3.6*Ns_Module*NumModules)  SampleTime=-1  HasFrameUpgradeWarning=on
  Rate Transition1 : RateTransition  InitialCondition=zeros(1,Ns_Module)  OutPortSampleTime=ts_system
  Cells : PMIOPort  Side=Left
  Bal_Cmd : Outport
  Sensor Values : Outport  Port=2
  tag scope: Balancing_Currents=global
  wires:
  Feedback Unit/1 -> Sensor Values/1
  Sensor_Values/1 -> Feedback Unit/1
  Bal_Cmd_Controller/1 -> Bal_Cmd/1, Rate Transition1/1
  Rate Transition1/1 -> Balancing_Circuit/1(Bal_Cmd_Controller)
  Balancing_Circuit/1(Balancing_Currents) -> [Balancing_Currents]
  connections:
  Balancing_Circuit/LConn1 -- Cells/RConn1

== system Copy_of_VTOLTiltrotor/Battery Management System/BMS/MIL/Controller ==
  Sensor_Values : Inport  OutDataTypeStr=Bus: Sensor_Values  BusOutputAsStruct=on
  State_Request : Inport  Port=2  OutDataTypeStr=Enum: SRE  PortDimensions=1
  BMS State Machine : Subsystem
  Balancing Logic : Subsystem
  Constant : Constant
  Current Calculations : Subsystem
  SOC Calculation : Subsystem
  Faults : Outport
  Charging_State : Outport  Port=2
  BMS_Controller_State : Outport  Port=3
  SOC : Outport  Port=4
  Discharge_Current_Limit : Outport  Port=5
  Charge_Current_Limit : Outport  Port=6
  Charge_Current_Req : Outport  Port=7
  Bal_Cmd : Outport  Port=8
  wires:
  SOC Calculation/1(SOC) -> SOC/1
  Current Calculations/1(Discharge_Current_Limit) -> Discharge_Current_Limit/1, BMS State Machine/1(Discharge_Current_Limit)
  BMS State Machine/2(Faults) -> Faults/1
  BMS State Machine/1(Charge_Current_Req) -> Charge_Current_Req/1
  Sensor_Values/1 -> Balancing Logic/2(Sensor_Values), SOC Calculation/2(Sensor_Values), BMS State Machine/4(Sensor_Values), Current Calculations/1(BMS_Input)
  BMS State Machine/4(BMS_State) -> BMS_Controller_State/1, Balancing Logic/1(BMS_State), SOC Calculation/1(BMS_State)
  Current Calculations/2(Charge_Current_Limit) -> Charge_Current_Limit/1, BMS State Machine/2(Charge_Current_Limit)
  Balancing Logic/1(Bal_Cmd) -> Bal_Cmd/1  "Bal_Cmd"
  State_Request/1 -> BMS State Machine/3(State_Request)
  Constant/1 -> BMS State Machine/5(Fault_Reset_Enable)
  BMS State Machine/3(Charging_State) -> Charging_State/1

== system Copy_of_VTOLTiltrotor/Battery Management System/Battery/Battery Pack/12-Cell ==
  Ambient_Temperature : Inport
  Short_Circuits : Inport  Port=2
  Controlled Temperature Source : fl_lib/Thermal/Thermal Sources/Controlled Temperature Source
      settings: LibrarySourceBlock=|
      | BatteryPack_lib/CellModule1TC/Controlled
      | Temperature Source
  Delay : Delay
  Faults : Subsystem
  Module1 : BatteryModuleLibrary_12Cells_lib/Module1  BatteryCapacityCell=27 A*hr  ExtrapolationMethodCell=simscape.enum.extrapolation.nearest  SOCBreakpointsCell=[0, .1, .25, .5, .75, .9, 1]  TemperatureBreakpointsCell=[278, 293, 313] K  OpenCircuitVoltageThermalCell=[3.49, 3.5, 3.51; 3.55, 3.57, 3.56; 3.62, 3.63, 3.64; 3.71, 3.71, 3.72; 3.91, 3.93, 3.94; 4.07, 4.08, 4.08; 4.19, 4.19, 4.19] V  VoltageRangeCell=[0, inf] V  ResistanceSOCBreakpointsCell=[0, .1, .25, .5, .75, .9, 1]  ResistanceTemperatureBreakpointsCell=[278, 293, 313] K  R0ThermalCell=[.0117, .0085, .009; .011, .0085, .009; .0114, .0087, .0092; .0107, .0082, .0088; .0107, .0083, .0091; .0113, .0085, .0089; .0116, .0085, .0089] Ohm  BatteryThermalMassCell=100 J/K  AmbientResistance=25 K/W  P=1  S=12  socCell_specify=off  socCell_priority=High  socCell=repmat(1, 12, 1)  socCell_nominal_specify=off  socCell_nominal_value=1  socCell_nominal_unit=1  numCycles_specify=off  numCycles_priority=High  numCycles=repmat(0, 12, 1)  numCycles_nominal_specify=off  numCycles_nominal_value=1  numCycles_nominal_unit=1  batteryVoltage_specify=off  batteryVoltage_priority=None  batteryVoltage=repmat(0, 12, 1) V  batteryVoltage_nominal_specify=off  batteryVoltage_nominal_value=1  batteryVoltage_nominal_unit=V  batteryCurrent_specify=off  batteryCurrent_priority=None  batteryCurrent=repmat(0, 12, 1) A  batteryCurrent_nominal_specify=off  batteryCurrent_nominal_value=1  batteryCurrent_nominal_unit=A  batteryTemperature_specify=off  batteryTemperature_priority=High  batteryTemperature=repmat(298.15, 12, 1) K  batteryTemperature_nominal_specify=off  batteryTemperature_nominal_value=1  batteryTemperature_nominal_unit=K  vParallelAssembly_specify=off  vParallelAssembly_priority=None  vParallelAssembly=repmat(0, 12, 1) V  vParallelAssembly_nominal_specify=off  vParallelAssembly_nominal_value=1  vParallelAssembly_nominal_unit=V  socParallelAssembly_specify=off  socParallelAssembly_priority=None  socParallelAssembly=repmat(1, 12, 1)  socParallelAssembly_nominal_specify=off  socParallelAssembly_nominal_value=1  socParallelAssembly_nominal_unit=1
      settings: InternalSimscapePortConfiguration="{\"Bottom\":[{\"id\":\"n\",\"label\":\"-\",\"type\":\"foundation.electrical.electrical\"}],\"Left\":[{\"id\":\"AmbH\",\"label\":\"AmbH\",\"type\":\"foundation.thermal.thermal\"}],\"Right\":[{\"id\":\"PositiveBus\",\"label\":\"+Bus\",\"type\":\"foundation.electrical.electrical\"},{\"id\":\"NegativeBus\",\"label\":\"-Bus\",\"type\":\"foundation.electrical.electrical\"}],\"Top\":[{\"id\":\"p\",\"label\":\"+\",\"type\":\"foundation.electrical.electrical\"}]}"
  PS-Simulink Converter : nesl_utility/PS-Simulink Converter  PhysicalDomain=network_engine_domain  SubClassName=ps_output  LeftPortType=input  RightPortType=output  PseudoPeriodic=off  Frequencies=[]  VectorFormat=inherit  Unit=inherit  AffineConversion=off
  Passive Balancing Interface1 : batt_lib/HIL/Passive Balancing Interface  balancingCircuitCount=12
      settings: InternalSimscapePortConfiguration="{\"Bottom\":[],\"Left\":[{\"id\":\"PositiveBus\",\"label\":\"+\",\"type\":\"foundation.electrical.electrical\"},{\"id\":\"NegativeBus\",\"label\":\"-\",\"type\":\"foundation.electrical.electrical\"}],\"Right\":[{\"id\":\"balancingCurrent\",\"label\":\"Ibat\",\"type\":\"input\"},{\"id\":\"balancingVoltage\",\"label\":\"Vbat\",\"type\":\"output\"}],\"Top\":[]}"
  Probe : SimscapeProbe  BoundBlock=12336  Variables={batteryTemperature, socParallelAssembly}
  Simulink-PS Converter : nesl_utility/Simulink-PS Converter  PhysicalDomain=network_engine_domain  SubClassName=ps_input  LeftPortType=input  RightPortType=output  PseudoPeriodic=off  Frequencies=[]  NoiseDistribution=none  NoiseParameters=[]  Unit=1  AffineConversion=off  FilteringAndDerivatives=provide  SimscapeFilterOrder=1  InputFilterTimeConstant=0.001  UdotUserProvided=0
  Simulink-PS Converter1 : nesl_utility/Simulink-PS Converter  PhysicalDomain=network_engine_domain  SubClassName=ps_input  LeftPortType=input  RightPortType=output  PseudoPeriodic=off  Frequencies=[]  NoiseDistribution=none  NoiseParameters=[]  Unit=1  AffineConversion=off  FilteringAndDerivatives=provide  SimscapeFilterOrder=1  InputFilterTimeConstant=0.001  UdotUserProvided=0
      settings: LibrarySourceBlock=|
      | BatteryPack_lib/CellModule1TC/Simulink-PS
      | Converter1
  Batt+ : PMIOPort  Side=Right
  Batt- : PMIOPort  Port=2  Side=Right
  Cells : PMIOPort  Port=3  Side=Right
  Cell_Voltages : Outport
  Cell_Temperatures : Outport  Port=2
  Cell_SOCs : Outport  Port=3
  wires:
  [Balancing_Currents] -> Delay/1
  Probe/1 -> Cell_Temperatures/1
  Probe/2 -> Cell_SOCs/1
  Delay/1 -> Simulink-PS Converter/1
  Short_Circuits/1 -> Faults/1(Short_Circuits)
  Ambient_Temperature/1 -> Simulink-PS Converter1/1
  PS-Simulink Converter/1 -> Cell_Voltages/1
  connections:
  Controlled Temperature Source/LConn1 -- Module1/LConn1
  Batt+/RConn1 -- Module1/LConn2
  Batt-/RConn1 -- Module1/RConn3
  Faults/RConn1 -- Passive Balancing Interface1/LConn1 -- Module1/RConn1
  Passive Balancing Interface1/RConn1 -- Simulink-PS Converter/RConn1
  Passive Balancing Interface1/RConn2 -- PS-Simulink Converter/LConn1
  Module1/RConn2 -- Faults/RConn3 -- Passive Balancing Interface1/LConn2
  Cells/RConn1 -- Faults/RConn2
  Simulink-PS Converter1/RConn1 -- Controlled Temperature Source/RConn1

== system Copy_of_VTOLTiltrotor/Battery Management System/Battery/Bypass/Bypass Values ==
  Input_Voltages : Inport
  Input_Temperatures : Inport  Port=2
  Broken_Wire : Inport  Port=3
  12-Cell : Subsystem  VariantControl=Ns_Module == 12
  Output_Voltages : Outport
  Output_Temperatures : Outport  Port=2
  wires:
  Input_Voltages/1 -> 12-Cell/1(Input_Voltages)
  Input_Temperatures/1 -> 12-Cell/2(Input_Temperatures)
  12-Cell/1(Output_Voltages) -> Output_Voltages/1
  12-Cell/2(Output_Temperatures) -> Output_Temperatures/1
  Broken_Wire/1 -> 12-Cell/3(Broken_Wire)

== system Copy_of_VTOLTiltrotor/Battery Management System/Battery/HW Interface/BCE - HIL ==
  Sensor_Values_Sim : Inport
  Add : Sum  Inputs=+
  Battery Cell Emulator : Subsystem
  Bus Creator : BusCreator  Inputs=4  OutDataTypeStr=Bus: Sensor_Values  NonVirtualBus=on
      settings: InheritFromInputs=off
  Data Type Conversion : DataTypeConversion  SaturateOnIntegerOverflow=off  RndMeth=Floor
  Shunt Emulator : Subsystem
  Temperature Emulator : Subsystem
  Cells_IN : PMIOPort  Side=Left
  Cells_OUT : PMIOPort  Port=2  Side=Right
  Sensor_Values_Real : Outport
  tag scope: Balancing_Currents=global
  wires:
  Sensor_Values_Sim/1 -> Battery Cell Emulator/1(Sensor_Values_Sim), Shunt Emulator/1(Sensor_Values_Sim), Temperature Emulator/1(Sensor_Values_Sim)
  Battery Cell Emulator/2(Cell_Voltages) -> Bus Creator/1, Add/1  "Cell_Voltages"
  Temperature Emulator/1(Cell_Temperatures) -> Bus Creator/2  "Cell_Temperatures"
  Add/1 -> Bus Creator/4  "Pack_Voltage"
  Bus Creator/1 -> Sensor_Values_Real/1
  Shunt Emulator/1(Pack_Current) -> Bus Creator/3  "Pack_Current"
  Battery Cell Emulator/1(Current_Values) -> Data Type Conversion/1
  Data Type Conversion/1 -> [Balancing_Currents]
  connections:
  Cells_OUT/RConn1 -- Cells_IN/RConn1

== system Copy_of_VTOLTiltrotor/Battery Management System/Battery/HW Interface/MIL ==
  Sensor_Values_Sim : Inport
  Cells_IN : PMIOPort  Side=Left
  Cells_OUT : PMIOPort  Port=2  Side=Right
  Sensor_Values_Real : Outport
  wires:
  Sensor_Values_Sim/1 -> Sensor_Values_Real/1
  connections:
  Cells_IN/RConn1 -- Cells_OUT/RConn1
